simulink model "Elevator_project (1)"  (R2020a)
settings: Solver=FixedStepAuto  StartTime=0.0  StopTime=inf  FixedStep=0.1  RelTol=1e-3
settings Model: EnablePacing=on  Creator=jatin  LastModifiedBy=jatin
settings RTWCC: GenCodeOnly=on  PackageGeneratedCodeAndArtifacts=on
settings GRTTargetCC: MatFileLogging=off
settings ConfigComp: DVMode=PropertyProving  DVMaxProcessTime=NaN  DVTestSuiteOptimization=Auto  DVDetectOutOfBounds=on

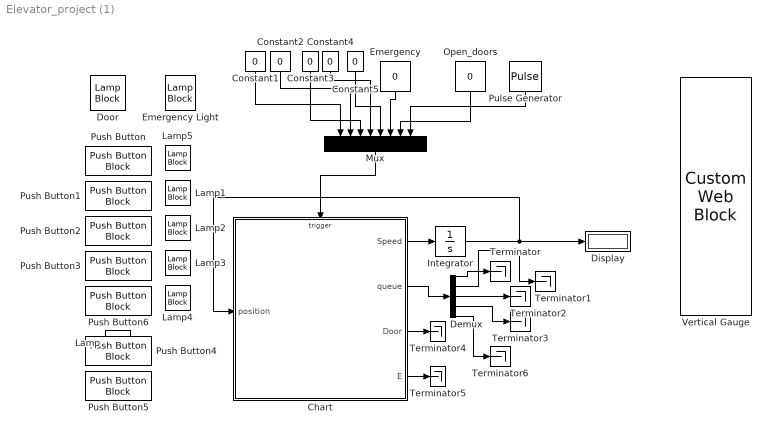
== system Elevator_project (1) ==
  Chart : Stateflow chart  TreatAsAtomicUnit=on
  Constant{1..5} (5 alike) : Constant  Value=0
  Demux : Demux  Outputs=5
  Display : Display
  Door : LampBlock
  Emergency : Constant  Value=0
  Emergency Light : LampBlock
  Integrator : Integrator
  Lamp{,1..5} (6 alike) : LampBlock
  Mux : Mux  Inputs=8
  Open_doors : Constant  Value=0
  Pulse Generator : DiscretePulseGenerator  PulseType=Time based  Period=1  PulseWidth=50
  Push Button : PushButtonBlock  ButtonText=floor0
  Push Button1 : PushButtonBlock  ButtonText=floor1
  Push Button2 : PushButtonBlock  ButtonText=floor2
  Push Button3 : PushButtonBlock  ButtonText=floor3
  Push Button4 : PushButtonBlock  ButtonText=Emergency
  Push Button5 : PushButtonBlock  ButtonText=Open_doors
  Push Button6 : PushButtonBlock  ButtonText=floor4
  Terminator{,1..6} (7 alike) : Terminator
  Vertical Gauge : CustomWebBlock  ShowInitialText=on  Configuration="{\"components\":[{\"name\":\"LinearScaleComponent\",\"settings\":{\"bounds\":{\"max\":4,\"min\":0,\"tickInterval\":\"auto\"},\"labelColor\":[250,245,199],\"labelFont\":{\"font\":\"Arial\",\"fontSize\":12},\"labelTransparency\":1,\"needleImage\":{\"size\":[21,75],\"src\":\"data:image\\/svg+xml;base64,PHN2ZyB4bWxucz0iaHR0cDovL3d3dy53My5vcmcvMjAwMC9zdmciIHhtbG5zOnhsaW5rPSJodHRwOi8vd3d3LnczLm9yZy8xOTk5L3hsaW5rIiB2aWV3Qm94PSIwIDAgMjEgNzUiPjxkZWZzPjxzdHlsZT4uY2xzLTF7ZmlsbDpub25lO30uY2xzLTJ7aXNvbGF0aW9uOmlzb2xhdGU7fS5jbHMtM3tjbGlwLXBhdGg6dXJsKCNjbGlwLXBhdGgpO30uY2xzLTR7b3BhY2l0eTowLjM7bWl4LWJsZW5kLW1vZGU6bXVsdGlwbHk7fS5jbHMtNXtmaWxsOiNlYjI2Mjk7fTwvc3R5bGU+PGNsaXBQYXRoIGlkPSJjbGlwLXBhdGgiIHRyYW5zZm9y ...(+1928 chars)\",\"srcOrientation\":\"horizontal\"},\"needleOffset\":[-0.01094391244870041,0],\"needleSize\":{\"height\":0.11960078534031414,\"width\":0.7589285714285714},\"position\":[0.015887605042016806,0.06986607142857143,0.8,0.9641544117647058],\"scaleColorSize\":0.24,\"scaleColors\":[],\"scaleColorsSize\":0.2,\"tickColor\":[250,245,200],\"tickTransparency\":1,\"valueBarColor\":[23,89,176],\"valueBarSize\":0.23,\"valueBarTransparency\":1}},{\"name\":\"BackgroundImageComponent\",\"settings\":{\"image\":{\"size\":[380,101],\"src\":\"data:image\\/svg+xml;base64,PHN2ZyB4bWxucz0iaHR0cDovL3d3dy53My5vcmcvMjAwMC9zdmciIHhtbG5zOnhsaW5rPSJodHRwOi8vd3d3LnczLm9yZy8xOTk5L3hsaW5rIiB2aWV3Qm94PSIwIDAgMzgwIDEwMSI+PGRlZnM+PHN0eWxlPi5jbHMtMXtmaWxsOnVybCgjbGluZWFyLWdyYWRpZW50KTt9LmNscy0ye2ZpbGw6dXJsKCNsaW5lYXItZ3JhZGllbnQtMik7fS5jbHMtM3tmaWxsOnVybCgjbGluZWFyLWdyYWRpZW50LTMpO308L3N0eWxlPjxsaW5lYXJHcmFkaWVudCBpZD0ibGluZWFyLWdyYWRpZW50IiB5MT0iNTAuNSIgeDI9IjM5OS4yOCIgeTI9IjUw ...(+2216 chars)\",\"srcOrientation\":\"horizontal\"},\"position\":[0,0,1,1],\"scaleMode\":\"0\"}}],\"settings\":{\"BindingType\":\"signal\",\"fixedAspectRatio\":\"on\",\"orientation\":\"vertical\"},\"type\":\"LinearGauge\"}"
  wires:
  Mux/1 -> Chart/Trigger
  Chart/2(queue) -> Demux/1
  Integrator/1 -> Chart/1(position), Display/1
  Constant1/1 -> Mux/1
  Constant2/1 -> Mux/2
  Constant3/1 -> Mux/3
  Constant4/1 -> Mux/4
  Constant5/1 -> Mux/5
  Emergency/1 -> Mux/6
  Open_doors/1 -> Mux/7
  Pulse Generator/1 -> Mux/8
  Chart/1(Speed) -> Integrator/1
  Chart/3(Door) -> Terminator4/1
  Chart/4(E) -> Terminator5/1
  Demux/5 -> Terminator6/1
  Demux/4 -> Terminator3/1
  Demux/3 -> Terminator2/1
  Demux/2 -> Terminator1/1
  Demux/1 -> Terminator/1

== stateflow chart Elevator_project (1)/Chart ==
  settings: executeAtInitialization=1
  state Init
    on floor0: queue(1)=1;
    on floor1: queue(2)=1;
    on floor2: queue(3)=1;
    on floor3: queue(4)=1;
    on floor4: queue(5)=1;
    on Open_doors: open_door=1;
    du: Error_check();
    state Up
      Speed=0.2;
      dir=1;
      floor_check();
    state Door
      Door=1;queue(dest)=0;
    state Idle_state
    state Emergency
      Speed=0;
    state Down
      Speed=-0.2;
      dir=-1;
      floor_check();
    Idle_state -> Door [order 2] : [current_floor()==1 || (open_door==1 && Speed==0)]{open_door=0;}
    Up -> Door [order 2] : [position>=dest-1.05]{Speed=0;}
    Idle_state -> Up [order 3] : [floor_check==1]
    Up -> Emergency [order 1] : Emergency{u=1;E=1;}
    Emergency -> Up [order 2] : Emergency[u==1]{u=0;E=0;}
    Door -> Door [order 2] : [open_door==1]{open_door=0;}
    (default) -> Idle_state
    Door -> Emergency [order 1] : Emergency{do=1;E=1;}
    Idle_state -> Emergency [order 1] : Emergency{i=1;E=1;}
    Emergency -> Door [order 3] : Emergency[do==1]{do=0;E=0;}
    Emergency -> Idle_state [order 1] : Emergency[i==1]{E=0;i=0;}
    Door -> Idle_state [order 3] : [after(5,tic)]{Door=0;}
    Down -> Door [order 1] : [position<=dest-0.8]{Speed=0;}
    Down -> Emergency [order 2] : Emergency{d=1;E=1;}
    Emergency -> Down [order 4] : Emergency[d==1]{d=0;E=0;}
    Idle_state -> Down [order 4] : [floor_check==0]
  (default) -> Init : {open_door=0;dest=1;Speed=0;queue(1)=0;Door=0;E=0;dir=0;i=0;u=0;d=0;do=0;}
  data: out function_output; o function_output; Speed output; dest local; queue output double size=[1 5]; Door output; E output; d local; do local; i local; u local; dir local; open_door local; position input
  events: floor0 input RISING_EDGE_EVENT; floor1 input RISING_EDGE_EVENT; floor2 input RISING_EDGE_EVENT; floor3 input RISING_EDGE_EVENT; floor4 input RISING_EDGE_EVENT; Emergency input RISING_EDGE_EVENT; Open_doors input RISING_EDGE_EVENT; tic input RISING_EDGE_EVENT
  function out = floor_check:
    | function out = floor_check
    | if dir>0
    |     if queue(2)&& position<1
    |         dest=2;
    |         out=1;  
    |     elseif queue(3) && position<2
    |         dest=3;
    |         out=1;
    |     elseif queue(4)&& position<3
    |         dest=4;
    |         out=1;
    |     elseif queue(5) && position~=4
    |         dest=5;
    |         out=1;
    |     else
    |         dir=0;
    |         out=-1;
    |     end
    | elseif dir<0
    |     if queue(4)&& position>3
    |         dest=4;
    |         out=0;    
    |     elseif queue(3)&& position>2
    |         dest=3;
    |         out=0;
    |     elseif queue(2)&& position>1
    |         dest=2;
    |         out=0;
    |     elseif queue(1)&& position~=0
    |         dest=1;
    |         out=0;
    |     else
    |         dir=0;
    |         out=-1;
    |     end
    | else
    |     if queue(1) && position~=0
    |         dest=1;
    |         out=0;
    |     elseif queue(2)
    |         if position>1
    |             dest=2;
    |             out=0;
    |         elseif position<1
    |             dest=2;
    |             out=1;
    |         else out=-1;
    |             dir=0;
    |         end
    |     elseif queue(3)
    |         if position>2
    |             dest=3;
    |             out=0;
    |         elseif position<2
    |             dest=3;
    |             out=1;
    |         else
    |             out=-1;
    |             dir=0;
    |         end
    |     elseif queue(4)
    |         if position>3
    |             dest=4;
    |             out=0;
    |         elseif position<3
    |             dest=4;
    |             out=1;
    |         else
    |             out=-1;
    |             dir=0;
    |         end
    |     elseif queue(5) && position~=4
    |         dest=5;
    |         out=1;
    |     else
    |         out=-1;
    |         dir=0;
    |     end
    | end
  function Error_check:
    | function Error_check
    | cur_pos=position;
    | if position>4.1 && position<0
    |     Speed=0;
    |     Door=0;
    | elseif (position==cur_pos + 0.5) || (position == cur_pos - 0.5)
    |      Speed=0;
    |      Door=0;
    | elseif (Speed>0 || Speed<0) && Door==1
    |     Speed=0;
    |     Door=0;
    | end
  function o=current_floor:
    | function o=current_floor
    | if dir==0
    |     if queue(1) && queue(2)==0 && queue(3)==0 && queue(4)==0 && queue(5)==0 && position<1 && position>=0
    |         o=1;
    |         dest=1;
    |     elseif queue(1)==0 && queue(2) && queue(3)==0 && queue(4)==0 && queue(5)==0 && position<2 && position>=1
    |         o=1;
    |         dest=2;
    |     elseif queue(1)==0 && queue(2)==0 && queue(3) && queue(4)==0 && queue(5)==0 && position<3 && position>=2
    |         o=1;
    |         dest=3;
    |     elseif queue(1)==0 && queue(2)==0 && queue(3)==0 && queue(4) && queue(5)==0 && position<4 && position>=3
    |         o=1;
    |         dest=4;
    |     elseif queue(1)==0 && queue(2)==0 && queue(3)==0 && queue(4)==0 && queue(5) && position>=4
    |         o=1;
    |         dest=5;
    |     else
    |         o=0;
    |     end
    | else
    |     o=0;
    | end
